simulink model "ModulesAndShaft"  (R2016a)
settings: Solver=VariableStepAuto  StartTime=0.0  StopTime=1  RelTol=1e-3
libraries: fl_lib x18, pe_lib x16, nesl_utility x13, dspstat3 x4, sdl_lib x1
settings Model: Creator=ugurm  LastModifiedBy=ugurm

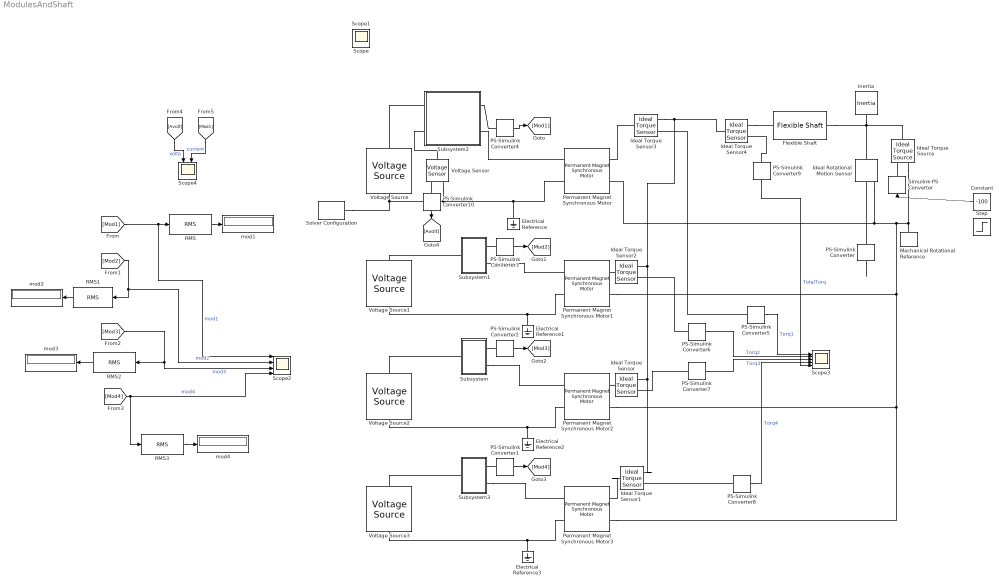
== system ModulesAndShaft ==
  Constant : Constant  Value=-100
  Electrical Reference{,1..3} (4 alike) : fl_lib/Electrical/Electrical Elements/Electrical Reference
  Flexible Shaft : sdl_lib/Couplings & Drives/Flexible Shaft  parameterization=1  shaft_stiffness=2e+5 N*m/rad  shaft_inertia=0.02 kg*m^2  shaft_construction=1  length=1 m  diameter_outer=0.075 m  diameter_inner=0.05 m  density=7.8e+3 kg/m^3  shear_modulus=7.93e+10 Pa  damping_ratio=0.01  n_segments=1  mu_visc=[ 0 0 ] N*m/(rad/s)  initial_deflection=0 rad  initial_velocity=0 rpm
  Ideal Rotational Motion Sensor : fl_lib/Mechanical/Mechanical Sensors/Ideal Rotational Motion Sensor  offset=0 rad
  Ideal Torque Sensor{,1..4} (5 alike) : fl_lib/Mechanical/Mechanical Sensors/Ideal Torque Sensor
  Ideal Torque Source : fl_lib/Mechanical/Mechanical Sources/Ideal Torque Source
  Inertia : fl_lib/Mechanical/Rotational Elements/Inertia  inertia=0.1 kg*m^2  w_specify=on  w_priority=High  w=0 rad/s  t_specify=on  t_priority=Low  t=0 N*m
  Mechanical Rotational Reference : fl_lib/Mechanical/Rotational Elements/Mechanical Rotational Reference
  PS-Simulink Converter{,1..10} (11 alike) : nesl_utility/PS-Simulink Converter  PhysicalDomain=network_engine_domain  SubClassName=ps_output  LeftPortType=input  RightPortType=output  PseudoPeriodic=off  Frequencies=[]  Unit=1  AffineConversion=off
  Permanent Magnet Synchronous Motor : pe_lib/Machines/Permanent Magnet Rotor/Permanent Magnet Synchronous Motor  nPolePairs=1  pm_flux_linkage=0.03 Wb  stator_param=1  Ld=0.00025 H  Lq=0.00019 H  L0=0.00016 H  Ls=0.0002 H  Lm=0.00002 H  Ms=0.00002 H  Rs=0.013 Ohm  initial_currents=[0.0, 0.0, 0.0] A  axes_param=2  angular_position0=0 deg  rotor_offset=- pi / 2 rad  shift_3ph=[nan, nan, nan] rad  sqrt2OverSqrt3=nan  oneOverSqrt2=nan  twoPiOver3=nan  Lmin=1e-9 H
  Permanent Magnet Synchronous Motor1 : pe_lib/Machines/Permanent Magnet Rotor/Permanent Magnet Synchronous Motor  nPolePairs=1  pm_flux_linkage=0.03 Wb  stator_param=1  Ld=0.00025 H  Lq=0.00019 H  L0=0.00016 H  Ls=0.0002 H  Lm=0.00002 H  Ms=0.00002 H  Rs=0.013 Ohm  initial_currents=[0.0, 0.0, 0.0] A  axes_param=2  angular_position0=90 deg  rotor_offset=- pi / 2 rad  shift_3ph=[nan, nan, nan] rad  sqrt2OverSqrt3=nan  oneOverSqrt2=nan  twoPiOver3=nan  Lmin=1e-9 H
  Permanent Magnet Synchronous Motor2 : pe_lib/Machines/Permanent Magnet Rotor/Permanent Magnet Synchronous Motor  nPolePairs=1  pm_flux_linkage=0.03 Wb  stator_param=1  Ld=0.00025 H  Lq=0.00019 H  L0=0.00016 H  Ls=0.0002 H  Lm=0.00002 H  Ms=0.00002 H  Rs=0.013 Ohm  initial_currents=[0.0, 0.0, 0.0] A  axes_param=2  angular_position0=180 deg  rotor_offset=- pi / 2 rad  shift_3ph=[nan, nan, nan] rad  sqrt2OverSqrt3=nan  oneOverSqrt2=nan  twoPiOver3=nan  Lmin=1e-9 H
  Permanent Magnet Synchronous Motor3 : pe_lib/Machines/Permanent Magnet Rotor/Permanent Magnet Synchronous Motor  nPolePairs=1  pm_flux_linkage=0.03 Wb  stator_param=1  Ld=0.00025 H  Lq=0.00019 H  L0=0.00016 H  Ls=0.0002 H  Lm=0.00002 H  Ms=0.00002 H  Rs=0.013 Ohm  initial_currents=[0.0, 0.0, 0.0] A  axes_param=2  angular_position0=270 deg  rotor_offset=- pi / 2 rad  shift_3ph=[nan, nan, nan] rad  sqrt2OverSqrt3=nan  oneOverSqrt2=nan  twoPiOver3=nan  Lmin=1e-9 H
  RMS{,1..3} (4 alike) : dspstat3/RMS  run=off  reset_popup=None  InputProcessing=Columns as channels (frame based)  directionMode=Each column  dimension=1
  Scope2 : Scope  NumInputPorts=4
  Scope3 : Scope  NumInputPorts=5
  Scope4 : Scope  NumInputPorts=2
  Simulink-PS Converter : nesl_utility/Simulink-PS Converter  PhysicalDomain=network_engine_domain  SubClassName=ps_input  LeftPortType=input  RightPortType=output  PseudoPeriodic=off  Frequencies=[]  NoiseDistribution=none  NoiseParameters=[]  Unit=1  AffineConversion=off  InputFiltering=off  SimscapeFilterOrder=1  InputFilterTimeConstant=0.001  UdotUserProvided=1
  Solver Configuration : nesl_utility/Solver Configuration  PhysicalDomain=network_engine_domain  SubClassName=solver  LeftPortType=input  RightPortType=generic  Accelerate=off  Tones=[]  Harmonics=[]  SimulateNoise=off  Profile=off  UseLocalSampling=off  EnableSwitchedLinearOptims=on  FrequencyDomain=off  UseCCode=off  RelTol=0.001  AbsTol=1e-06  MinStep=1e-09  ToWorkspace=off  RevertToSquareIcSolve=off  NumHomotopyIterations=100  PhasorMode=off  PhasorModeNumHarmonics=1  OverrideAbsTol=off  DoDC=off  ResidualTolerance=1e-09  UseLocalSolver=on  LocalSolverChoice=NE_BACKWARD_EULER_ADVANCER  LocalSolverSampleTime=1e-06  DoFixedCost=on  MaxNonlinIter=3  MaxModeIter=2  LinearAlgebra=Sparse  DelaysMemoryBudget=1024  AutomaticFiltering=on  FilteringTimeConstant=0.001
  Step : Step  Time=0.1  After=100  SampleTime=0
  Subsystem : Subsystem
  Subsystem1 : Subsystem
  Subsystem2 : Subsystem
  Subsystem3 : Subsystem
  Voltage Sensor : fl_lib/Electrical/Electrical Sensors/Voltage Sensor
  Voltage Source{,1..3} (4 alike) : pe_lib/Sources/Voltage Source  vline_rms=sqrt(3) * 220 V  shift=0 deg  freq=50 Hz  harmonic_option=0  harmonic_orders=[5.0, 7.0, 11.0, 13.0]  harmonic_ratios=[0.1, 0.1, 0.1, 0.1]
  mod{1..4} (4 alike) : Display
  Scope : Scope
  Scope1 : Scope
  wires:
  PS-Simulink Converter/1 -> ?
  PS-Simulink Converter4/1 -> [Mod1]
  PS-Simulink Converter3/1 -> [Mod2]
  PS-Simulink Converter1/1 -> [Mod4]
  PS-Simulink Converter2/1 -> [Mod3]
  [Mod1] -> RMS/1, Scope2/1  "mod1"
  [Mod2] -> RMS1/1, Scope2/2  "mod2"
  [Mod3] -> Scope2/3, RMS2/1  "mod3"
  [Mod4] -> Scope2/4, RMS3/1  "mod4"
  RMS3/1 -> mod4/1
  RMS2/1 -> mod3/1
  RMS/1 -> mod1/1
  RMS1/1 -> mod2/1
  PS-Simulink Converter5/1 -> Scope3/1  "Torq1"
  PS-Simulink Converter6/1 -> Scope3/2  "Torq2"
  PS-Simulink Converter7/1 -> Scope3/3  "Torq3"
  PS-Simulink Converter8/1 -> Scope3/4  "Torq4"
  PS-Simulink Converter9/1 -> Scope3/5  "TotalTorq"
  Constant/1 -> Simulink-PS Converter/1
  PS-Simulink Converter10/1 -> [Avolt]
  [Avolt] -> Scope4/1  "volta"
  [Mod1] -> Scope4/2  "current"
  connections:
  Voltage Source/LConn1 -- Voltage Sensor/RConn2 -- Electrical Reference/LConn1 -- Permanent Magnet Synchronous Motor/LConn2 -- Solver Configuration/RConn1
  Ideal Torque Source/RConn2 -- Permanent Magnet Synchronous Motor2/RConn2 -- Permanent Magnet Synchronous Motor3/RConn2 -- Permanent Magnet Synchronous Motor1/RConn2 -- Permanent Magnet Synchronous Motor/RConn2 -- Ideal Rotational Motion Sensor/RConn1 -- Mechanical Rotational Reference/LConn1
  Simulink-PS Converter/RConn1 -- Ideal Torque Source/RConn1
  Voltage Source1/LConn1 -- Electrical Reference1/LConn1 -- Permanent Magnet Synchronous Motor1/LConn2
  PS-Simulink Converter/LConn1 -- Ideal Rotational Motion Sensor/RConn2
  Flexible Shaft/RConn1 -- Ideal Rotational Motion Sensor/LConn1 -- Inertia/LConn1 -- Ideal Torque Source/LConn1
  Permanent Magnet Synchronous Motor2/LConn2 -- Electrical Reference2/LConn1 -- Voltage Source2/LConn1
  Permanent Magnet Synchronous Motor3/LConn2 -- Electrical Reference3/LConn1 -- Voltage Source3/LConn1
  Subsystem/LConn1 -- Voltage Source2/RConn1
  Subsystem/RConn2 -- Permanent Magnet Synchronous Motor2/LConn1
  Subsystem1/LConn1 -- Voltage Source1/RConn1
  Subsystem1/RConn2 -- Permanent Magnet Synchronous Motor1/LConn1
  Subsystem2/RConn2 -- Permanent Magnet Synchronous Motor/LConn1
  Subsystem2/LConn1 -- Voltage Source/RConn1
  Subsystem3/RConn2 -- Permanent Magnet Synchronous Motor3/LConn1
  Subsystem3/LConn1 -- Voltage Source3/RConn1
  PS-Simulink Converter1/LConn1 -- Subsystem3/RConn1
  PS-Simulink Converter2/LConn1 -- Subsystem/RConn1
  PS-Simulink Converter3/LConn1 -- Subsystem1/RConn1
  PS-Simulink Converter4/LConn1 -- Subsystem2/RConn1
  Ideal Torque Sensor/LConn1 -- Permanent Magnet Synchronous Motor2/RConn1
  Ideal Torque Sensor1/LConn1 -- Permanent Magnet Synchronous Motor3/RConn1
  Permanent Magnet Synchronous Motor/RConn1 -- Ideal Torque Sensor3/LConn1
  PS-Simulink Converter5/LConn1 -- Ideal Torque Sensor3/RConn2
  PS-Simulink Converter6/LConn1 -- Ideal Torque Sensor2/RConn2
  PS-Simulink Converter7/LConn1 -- Ideal Torque Sensor/RConn2
  PS-Simulink Converter8/LConn1 -- Ideal Torque Sensor1/RConn2
  Permanent Magnet Synchronous Motor1/RConn1 -- Ideal Torque Sensor2/LConn1
  Ideal Torque Sensor3/RConn1 -- Ideal Torque Sensor1/RConn1 -- Ideal Torque Sensor/RConn1 -- Ideal Torque Sensor2/RConn1 -- Ideal Torque Sensor4/LConn1
  Ideal Torque Sensor4/RConn1 -- Flexible Shaft/LConn1
  PS-Simulink Converter9/LConn1 -- Ideal Torque Sensor4/RConn2
  Voltage Sensor/LConn1 -- Subsystem2/LConn2
  PS-Simulink Converter10/LConn1 -- Voltage Sensor/RConn1

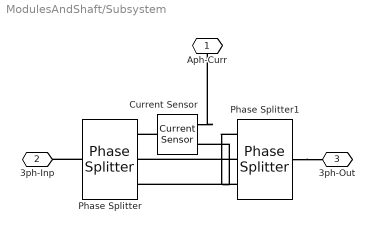
== system ModulesAndShaft/Subsystem ==
  Current Sensor : fl_lib/Electrical/Electrical Sensors/Current Sensor
  Phase Splitter : pe_lib/Connections/Phase Splitter
  Phase Splitter1 : pe_lib/Connections/Phase Splitter
  Aph-Curr : PMIOPort  Port=1  Side=Right
  3ph-Inp : PMIOPort  Port=2  Side=Left
  3ph-Out : PMIOPort  Port=3  Side=Right
  connections:
  Phase Splitter1/LConn1 -- 3ph-Out/RConn1
  Phase Splitter/LConn1 -- 3ph-Inp/RConn1
  Phase Splitter1/RConn1 -- Current Sensor/RConn2
  Current Sensor/LConn1 -- Phase Splitter/RConn1
  Current Sensor/RConn1 -- Aph-Curr/RConn1
  Phase Splitter1/RConn3 -- Phase Splitter/RConn3
  Phase Splitter1/RConn2 -- Phase Splitter/RConn2

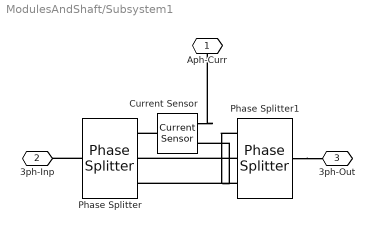
== system ModulesAndShaft/Subsystem1 ==
  Current Sensor : fl_lib/Electrical/Electrical Sensors/Current Sensor
  Phase Splitter : pe_lib/Connections/Phase Splitter
  Phase Splitter1 : pe_lib/Connections/Phase Splitter
  Aph-Curr : PMIOPort  Port=1  Side=Right
  3ph-Inp : PMIOPort  Port=2  Side=Left
  3ph-Out : PMIOPort  Port=3  Side=Right
  connections:
  Phase Splitter1/LConn1 -- 3ph-Out/RConn1
  Phase Splitter/LConn1 -- 3ph-Inp/RConn1
  Phase Splitter1/RConn1 -- Current Sensor/RConn2
  Current Sensor/LConn1 -- Phase Splitter/RConn1
  Current Sensor/RConn1 -- Aph-Curr/RConn1
  Phase Splitter1/RConn3 -- Phase Splitter/RConn3
  Phase Splitter1/RConn2 -- Phase Splitter/RConn2

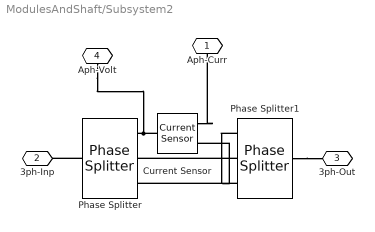
== system ModulesAndShaft/Subsystem2 ==
  Current Sensor : fl_lib/Electrical/Electrical Sensors/Current Sensor
  Phase Splitter : pe_lib/Connections/Phase Splitter
  Phase Splitter1 : pe_lib/Connections/Phase Splitter
  Aph-Curr : PMIOPort  Port=1  Side=Right
  3ph-Inp : PMIOPort  Port=2  Side=Left
  3ph-Out : PMIOPort  Port=3  Side=Right
  Aph-Volt : PMIOPort  Port=4  Side=Left
  connections:
  Phase Splitter1/LConn1 -- 3ph-Out/RConn1
  Phase Splitter/LConn1 -- 3ph-Inp/RConn1
  Phase Splitter1/RConn1 -- Current Sensor/RConn2
  Current Sensor/LConn1 -- Aph-Volt/RConn1 -- Phase Splitter/RConn1
  Current Sensor/RConn1 -- Aph-Curr/RConn1
  Phase Splitter1/RConn3 -- Phase Splitter/RConn3
  Phase Splitter1/RConn2 -- Phase Splitter/RConn2

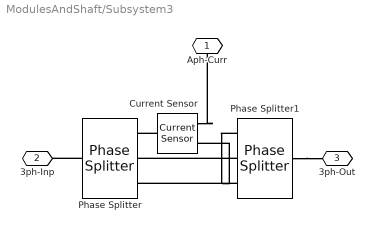
== system ModulesAndShaft/Subsystem3 ==
  Current Sensor : fl_lib/Electrical/Electrical Sensors/Current Sensor
  Phase Splitter : pe_lib/Connections/Phase Splitter
  Phase Splitter1 : pe_lib/Connections/Phase Splitter
  Aph-Curr : PMIOPort  Port=1  Side=Right
  3ph-Inp : PMIOPort  Port=2  Side=Left
  3ph-Out : PMIOPort  Port=3  Side=Right
  connections:
  Phase Splitter1/LConn1 -- 3ph-Out/RConn1
  Phase Splitter/LConn1 -- 3ph-Inp/RConn1
  Phase Splitter1/RConn1 -- Current Sensor/RConn2
  Current Sensor/LConn1 -- Phase Splitter/RConn1
  Current Sensor/RConn1 -- Aph-Curr/RConn1
  Phase Splitter1/RConn3 -- Phase Splitter/RConn3
  Phase Splitter1/RConn2 -- Phase Splitter/RConn2
